simulink model "dinamicadosistema"  (R2015a)
settings: Solver=ode45  StartTime=0.0  StopTime=10.0  RelTol=1e-3
values from neighbouring files (symbols this model uses):
  b = 0.025    [lab2.m]
  dy0 = 0    [lab2.m]
  y0 = 1    [lab2.m]
settings Model: Creator=Diogo  LastModifiedBy=Diogo

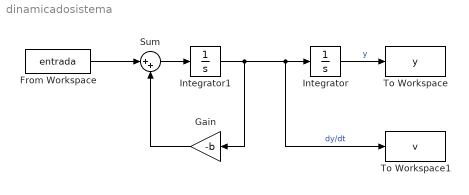
== system dinamicadosistema ==
  From Workspace : FromWorkspace  VariableName=entrada  SampleTime=0
  Gain : Gain  Gain=-b
  Integrator : Integrator  InitialCondition=y0
  Integrator1 : Integrator  InitialCondition=dy0
  Sum : Sum  Inputs=|++
  To Workspace : ToWorkspace  VariableName=y  SampleTime=-1
  To Workspace1 : ToWorkspace  VariableName=v  SampleTime=-1
  wires:
  From Workspace/1 -> Sum/1
  Sum/1 -> Integrator1/1
  Integrator1/1 -> To Workspace1/1, Integrator/1, Gain/1  "dy/dt"
  Integrator/1 -> To Workspace/1  "y"
  Gain/1 -> Sum/2
